simulink model "lvrotor5"  (Simulink 7.1)
settings: Solver=ode45  StartTime=0.0  StopTime=10.0  RelTol=1e-3
values from neighbouring files (symbols this model uses):
  c1 = 1.5    [find_bigvalue.m]    (also in find_bigvalue1.m)
undefined symbols (not defined in the file or in its folder): c2, c3, c4, c5, c6
settings Model: Creator=lv  LastModifiedBy=lv

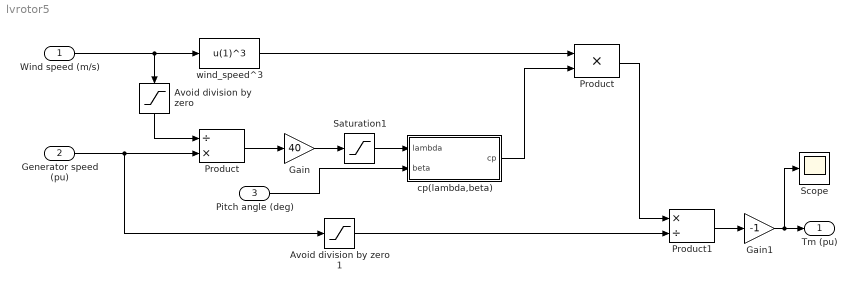
== system lvrotor5 ==
  Wind speed (m/s) : Inport  OutDataType=sfix(16)  OutScaling=2^0
  Generator speed (pu) : Inport  Port=2  OutDataType=sfix(16)  OutScaling=2^0
  Pitch angle (deg) : Inport  Port=3  OutDataType=sfix(16)  OutScaling=2^0
  "Avoid division by zero " : Saturate  Orientation=down  UpperLimit=1e6  LowerLimit=1e-6  OutDataType=sfix(16)  OutScaling=2^0
  Avoid division by zero 1 : Saturate  UpperLimit=1e6  LowerLimit=1e-6  OutDataType=sfix(16)  OutScaling=2^0
  Gain : Gain  Gain=40  ParameterDataType=sfix(16)  ParameterScaling=2^0  OutDataType=sfix(16)  OutScaling=2^0
  Gain1 : Gain  Gain=-1  ParameterDataType=sfix(16)  ParameterScaling=2^0  OutDataType=sfix(16)  OutScaling=2^0  SaturateOnIntegerOverflow=on  OutDataTypeStr=Inherit: Same as input  ParamDataTypeStr=Inherit: Same as input
  Product : Product  Inputs=/*  OutDataType=sfix(16)  OutScaling=2^0  SaturateOnIntegerOverflow=on  OutDataTypeStr=Inherit: Same as first input
  "Product " : Product  OutDataType=sfix(16)  OutScaling=2^0  SaturateOnIntegerOverflow=on  OutDataTypeStr=Inherit: Same as first input
  Product1 : Product  Inputs=*/  OutDataType=sfix(16)  OutScaling=2^0  SaturateOnIntegerOverflow=on  OutDataTypeStr=Inherit: Same as first input
  Saturation1 : Saturate  UpperLimit=inf  LowerLimit=1e-6  OutDataType=sfix(16)  OutScaling=2^0
  Scope : Scope
  cp(lambda,beta) : Subsystem
  wind_speed^3 : Fcn  Expr=u(1)^3
  Tm (pu) : Outport  OutDataType=sfix(16)  OutScaling=2^0
  wires:
  Gain1/1 -> Tm (pu)/1, Scope/1
  Product1/1 -> Gain1/1
  Avoid division by zero 1/1 -> Product1/2
  "Product "/1 -> Product1/1
  Saturation1/1 -> cp(lambda,beta)/1(lambda)
  Gain/1 -> Saturation1/1
  cp(lambda,beta)/1(cp) -> "Product "/2
  Pitch angle (deg)/1 -> cp(lambda,beta)/2(beta)
  Product/1 -> Gain/1
  "Avoid division by zero "/1 -> Product/1
  Generator speed (pu)/1 -> Product/2, Avoid division by zero 1/1
  wind_speed^3/1 -> "Product "/1
  Wind speed (m/s)/1 -> wind_speed^3/1, "Avoid division by zero "/1

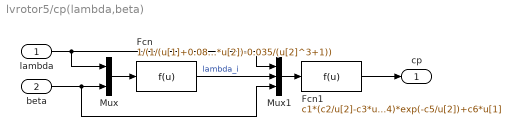
== system lvrotor5/cp(lambda,beta) ==
  lambda : Inport  OutDataType=sfix(16)  OutScaling=2^0
  beta : Inport  Port=2  OutDataType=sfix(16)  OutScaling=2^0
  Fcn : Fcn  Expr=1/(1/(u[1]+0.08*u[2])-0.035/(u[2]^3+1))
  Fcn1 : Fcn  Expr=c1*(c2/u[2]-c3*u[3]-c4)*exp(-c5/u[2])+c6*u[1]
  Mux : Mux  Inputs=2
  Mux1 : Mux  Inputs=3
  cp : Outport  OutDataType=sfix(16)  OutScaling=2^0
  wires:
  Fcn/1 -> Mux1/2  "lambda_i"
  Fcn1/1 -> cp/1
  lambda/1 -> Mux1/1, Mux/1
  Mux1/1 -> Fcn1/1
  beta/1 -> Mux1/3, Mux/2
  Mux/1 -> Fcn/1
